simulink model "Zadatak1b_Dahlin_PID"  (R2020b)
settings: Solver=VariableStepAuto  StartTime=0.0  StopTime=50.0  RelTol=1e-3
settings Model: Creator=user  LastModifiedBy=user

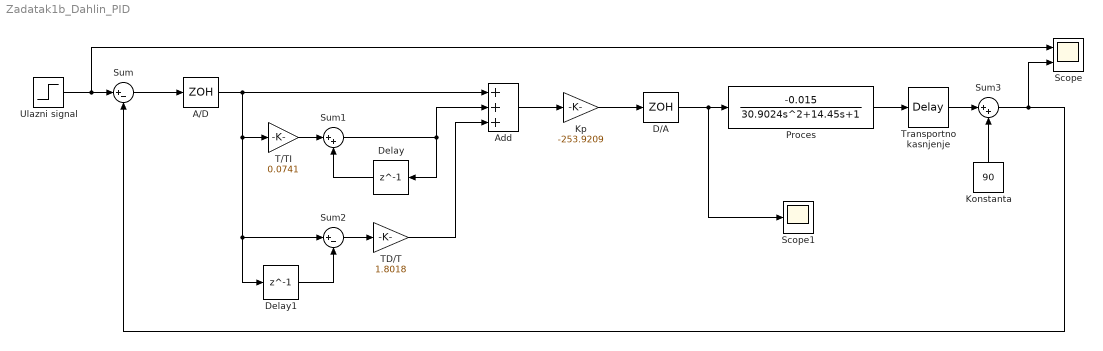
== system Zadatak1b_Dahlin_PID ==
  A/D : ZeroOrderHold
  Add : Sum  Inputs=+++
  D/A : ZeroOrderHold
  Delay : Delay  DelayLength=1
  Delay1 : Delay  DelayLength=1
  Konstanta : Constant  Value=90
  Kp : Gain  Gain=-253.9209
  Proces : TransferFcn  Numerator=[-0.015]  Denominator=[30.9024 14.45 1]
  Scope : Scope  NumInputPorts=2
  Scope1 : Scope
  Sum : Sum  Inputs=|+-
  Sum1 : Sum  Inputs=|++
  Sum2 : Sum  Inputs=|+-
  Sum3 : Sum  Inputs=|++
  T/TI : Gain  Gain=0.0741
  TD/T : Gain  Gain=1.8018
  Transportno kasnjenje : TransportDelay
  Ulazni signal : Step  Time=5  Before=90  After=80  SampleTime=0
  wires:
  D/A/1 -> Scope1/1, Proces/1
  Sum2/1 -> TD/T/1
  Proces/1 -> Transportno kasnjenje/1
  Transportno kasnjenje/1 -> Sum3/1
  Sum/1 -> A/D/1
  T/TI/1 -> Sum1/1
  Delay/1 -> Sum1/2
  Delay1/1 -> Sum2/2
  A/D/1 -> Sum2/1, Delay1/1, T/TI/1, Add/1
  Sum3/1 -> Sum/2, Scope/2
  Kp/1 -> D/A/1
  Add/1 -> Kp/1
  Konstanta/1 -> Sum3/2
  Ulazni signal/1 -> Scope/1, Sum/1
  TD/T/1 -> Add/3
  Sum1/1 -> Delay/1, Add/2
